simulink model "ModuladorDeTension"  (R2023b)
settings: Solver=VariableStepAuto  StartTime=0.0  StopTime=10.0  RelTol=1e-3
settings Model: Creator=gonza  LastModifiedBy=tomas

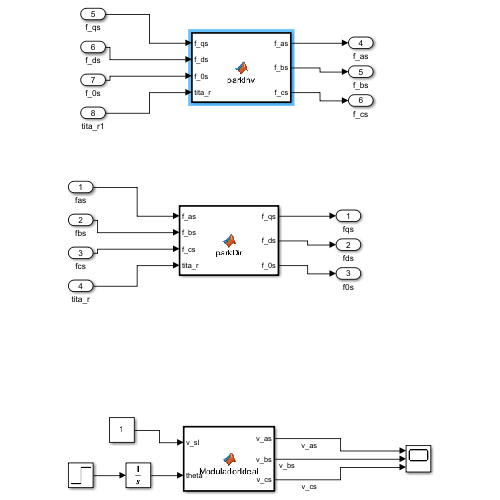
[thumbnail: Simulink's stored preview of the top-level diagram]
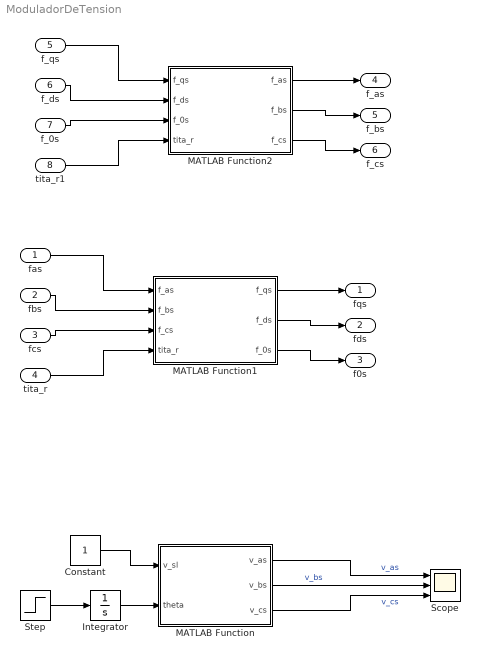
== system ModuladorDeTension ==
  fas : Inport
  fbs : Inport  Port=2
  fcs : Inport  Port=3
  tita_r : Inport  Port=4
  f_qs : Inport  Port=5
  f_ds : Inport  Port=6
  f_0s : Inport  Port=7
  tita_r1 : Inport  Port=8
  Constant : Constant
  Integrator : Integrator
  MATLAB Function : MATLAB Function  TreatAsAtomicUnit=on
  MATLAB Function1 : MATLAB Function  TreatAsAtomicUnit=on
  MATLAB Function2 : MATLAB Function  TreatAsAtomicUnit=on
  Scope : Scope  NumInputPorts=3
  Step : Step  SampleTime=0
  fqs : Outport
  fds : Outport  Port=2
  f0s : Outport  Port=3
  f_as : Outport  Port=4
  f_bs : Outport  Port=5
  f_cs : Outport  Port=6
  wires:
  MATLAB Function/1(v_as) -> Scope/1  "v_as"
  MATLAB Function/2(v_bs) -> Scope/2  "v_bs"
  MATLAB Function/3(v_cs) -> Scope/3  "v_cs"
  Constant/1 -> MATLAB Function/1(v_sl)
  Step/1 -> Integrator/1
  Integrator/1 -> MATLAB Function/2(theta)
  fas/1 -> MATLAB Function1/1(f_as)
  fbs/1 -> MATLAB Function1/2(f_bs)
  fcs/1 -> MATLAB Function1/3(f_cs)
  tita_r/1 -> MATLAB Function1/4(tita_r)
  MATLAB Function1/3(f_0s) -> f0s/1
  MATLAB Function1/2(f_ds) -> fds/1
  MATLAB Function1/1(f_qs) -> fqs/1
  MATLAB Function2/3(f_cs) -> f_cs/1
  f_0s/1 -> MATLAB Function2/3(f_0s)
  f_ds/1 -> MATLAB Function2/2(f_ds)
  MATLAB Function2/1(f_as) -> f_as/1
  f_qs/1 -> MATLAB Function2/1(f_qs)
  MATLAB Function2/2(f_bs) -> f_bs/1
  tita_r1/1 -> MATLAB Function2/4(tita_r)

== matlab function ModuladorDeTension/MATLAB Function1 ==
  data: f_as input; f_qs output; f_bs input; f_cs input; tita_r input; f_ds output; f_0s output
function [f_qs, f_ds, f_0s] = parkDir(f_as,f_bs,f_cs,tita_r)

answer = 2/3 * [cos(tita_r), cos(tita_r - 2*pi/3), cos(tita_r + 2*pi/3);
         sin(tita_r), sin(tita_r - 2*pi/3), sin(tita_r + 2*pi/3);
         1/2, 1/2, 1/2] * [f_as;f_bs;f_cs];

f_qs = answer(1);
f_ds = answer(2);
f_0s = answer(3);

== matlab function ModuladorDeTension/MATLAB Function ==
  data: v_sl input; v_as output; theta input; v_bs output; v_cs output
function [v_as,v_bs,v_cs] = ModuladorIdeal(v_sl,theta)
v_as=sqrt(2/3)*v_sl*cos(theta);
v_bs=sqrt(2/3)*v_sl*cos(theta-(2*pi)/(3));
v_cs=sqrt(2/3)*v_sl*cos(theta+(2*pi)/(3));

== matlab function ModuladorDeTension/MATLAB Function2 ==
  data: f_qs input; f_as output; f_ds input; f_0s input; tita_r input; f_bs output; f_cs output
function [f_as, f_bs, f_cs] = parkInv(f_qs,f_ds,f_0s,tita_r)

answer = [cos(tita_r), sin(tita_r), 1;
         cos(tita_r - 2*pi/3), sin(tita_r - 2*pi/3), 1;
         cos(tita_r + 2*pi/3), sin(tita_r + 2*pi/3), 1] * [f_qs;f_ds;f_0s]; 

f_as = answer(1);
f_bs = answer(2);
f_cs = answer(3);
